simulink model "dpsk"  (R2023b)
settings: Solver=VariableStepAuto  StartTime=0.0  StopTime=280  RelTol=1e-3
libraries: commdigbbndpm3 x2, commchan3 x1, commsink2 x1, simulink x1
settings Model: Creator=Vibha  LastModifiedBy=udaip
settings SolverCC: AlgebraicLoopSolver=TrustRegion
settings DataIOCC: ReturnWorkspaceOutputs=off
settings DebuggingCC: UnconnectedInputMsg=warning  UnconnectedOutputMsg=warning  UnconnectedLineMsg=warning  ArithmeticOperatorsInVariantConditions=warning
settings ModelReferenceCC: EnableRefExpFcnMdlSchedulingChecks=on
settings SFSimCC: SimUseLocalCustomCode=off  CustomCodeUndefinedFunction=UseInterfaceOnly
settings RTWCC: RTWUseLocalCustomCode=off
settings CodeAppCC: StateflowObjectComments=on

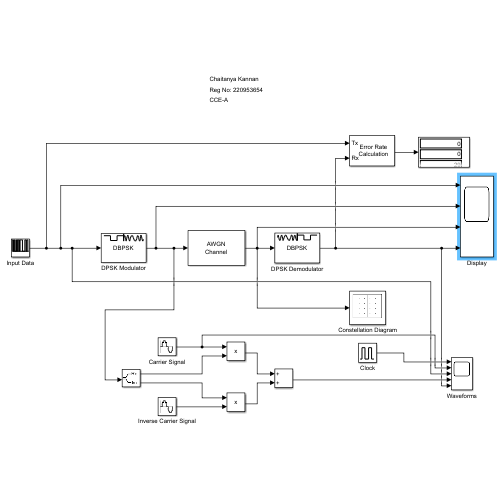
[thumbnail: Simulink's stored preview of the top-level diagram]
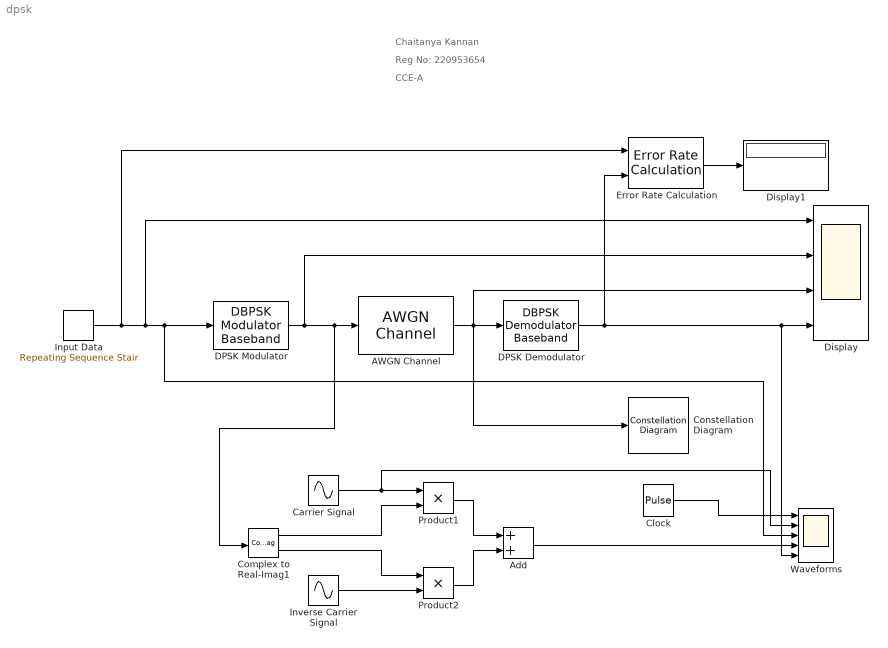
== system dpsk ==
  note: Chaitanya Kannan
  note: CCE-A
  note: Reg No: 220953654
  AWGN Channel : commchan3/AWGN Channel  LegacyMode=on  NoiseMethod="Signal to noise ratio  (SNR)"  noiseMode="Signal to noise ratio  (SNR)"  EbNo=10  EsNo=10  SNR=10  BitsPerSymbol=2  SignalPower=1  SamplesPerSymbol=1  SymbolPeriod=1  VarianceSource=Parameter  Variance=1  RandomStream=Global stream  Seed=67  SimulateUsing=Code generation
  Add : Sum
  Carrier Signal : Sin  Frequency=0.8*pi  SampleTime=0.001  VectorParams1D=off
  Clock : DiscretePulseGenerator  PulseType=Time based  Period=10  PulseWidth=50
  Complex to Real-Imag1 : ComplexToRealImag
  Constellation Diagram : ConstellationDiagram  WindowPosition=[1.000000,41.000000,1504.000000,940.000000,]  ScopeFrameLocation=window  SymbolsToDisplaySource=Property  SymbolsToDisplay=1000  XLimits=[-1.375,1.9081475113707103]  MaximizeAxes=off  DefaultConfigurationName=comm.scopes.ConstellationDiagramBlockCfg
  DPSK Demodulator : commdigbbndpm3/DBPSK Demodulator Baseband  Ph=0  outDtype=Inherit via internal rule
  DPSK Modulator : commdigbbndpm3/DBPSK Modulator Baseband  Ph=0  outDtype=double
  Display : Scope  NumInputPorts=4
  Display1 : Display
  Error Rate Calculation : commsink2/Error Rate Calculation  N=0  st_delay=0  cp_mode=Entire frame  subframe=[]  PMode=Port  WsName=ErrorVec  RsMode2=off  stop=off  numErr=100  maxBits=1e6
      settings: LibrarySourceBlock=|
      | commhdlsink/Error Rate
      | Calculation
  Input Data : simulink/Sources/Repeating Sequence Stair  OutValues=[1,1,0,1,0,0,1,0,1,0,1,1,0,1,1,1,1,1,0,0,0,0,1,1,0,1,1,0]  tsamp=10  OutMin=[]  OutMax=[]  OutDataTypeStr=double  OutputDataTypeScalingMode=double  OutDataType=fixdt(0,8)  ConRadixGroup=Best Precision: Vector-wise  OutScaling=2^-12
      settings: LibrarySourceBlock=|
      | hdlsllib/Sources/Repeating
      | Sequence
      | Stair
  Inverse Carrier Signal : Sin  Frequency=0.8*pi  Phase=pi/2  SampleTime=0.001  VectorParams1D=off
  Product1 : Product
  Product2 : Product
  Waveforms : Scope  NumInputPorts=5
  wires:
  AWGN Channel/1 -> DPSK Demodulator/1, Constellation Diagram/1, Display/3
  DPSK Demodulator/1 -> Display/4, Waveforms/5, Error Rate Calculation/2
  DPSK Modulator/1 -> Complex to Real-Imag1/1, AWGN Channel/1, Display/2
  Product1/1 -> Add/1
  Product2/1 -> Add/2
  Complex to Real-Imag1/2 -> Product2/1
  Complex to Real-Imag1/1 -> Product1/2
  Input Data/1 -> Error Rate Calculation/1, Waveforms/3, DPSK Modulator/1, Display/1
  Carrier Signal/1 -> Waveforms/2, Product1/1
  Inverse Carrier Signal/1 -> Product2/2
  Add/1 -> Waveforms/4
  Clock/1 -> Waveforms/1
  Error Rate Calculation/1 -> Display1/1
